simulink model "sgMdl_IO337_AnalogLoopback"  (R2024b)
settings: Solver=FixedStepAuto  StartTime=0.0  StopTime=inf  RelTol=1e-3
undefined symbols (not defined in the file): IO336, IO3xx, Pull, pull, up
libraries: speedgoatlib_fpga_analog_io x3, slrealtimeloglib x2, speedgoatlib_fpga x1
Description:
  | IO337 - Analog Loopback
settings Model: ModifiedByFormat=Speedgoat  SimulationMode=external  ExtModeTrigDuration=100000  Creator=Speedgoat  LastModifiedBy=Speedgoat
settings SolverCC: ConcurrentTasks=on  PositivePriorityOrder=on
settings DataIOCC: SaveFormat=StructureWithTime
settings OptimizationCC: BlockReduction=off  OptimizeBlockIOStorage=off  BufferReuse=off  ReuseModelBlockBuffer=off
settings DebuggingCC: UnderspecifiedInitializationDetection=Classic  MergeDetectMultiDrivingBlocksExec=none  TasksWithSamePriorityMsg=none
settings HardwareCC: ProdBitPerLong=64  ProdLongLongMode=on  ProdHWDeviceType=Intel->x86-64 (Linux 64)
settings ModelReferenceCC: EnableRefExpFcnMdlSchedulingChecks=on  PropagateSignalLabelsOutOfModel=off
settings RTWCC: Description=Speedgoat Real-Time Target Machine  SystemTargetFile=speedgoat.tlc  TemplateMakefile=slrealtime_default_tmf  PostCodeGenCommand=sg.model.build.makeCfg(bdroot, buildInfo);  Toolchain=Simulink Real-Time Toolchain  BuildConfiguration=Faster Runs  TargetLang=C++  GPUComputeCapability=3.5
settings SimulinkRealTimeTargetCC: SubcomponentCodeInterfacePackaging=Reusable function  InstructionSetFMA=off  LogToMDFFile=off  SLRTFileLogMaxRuns=10
settings ConfigComp: CovBoundaryAbsTol=1.0e-5

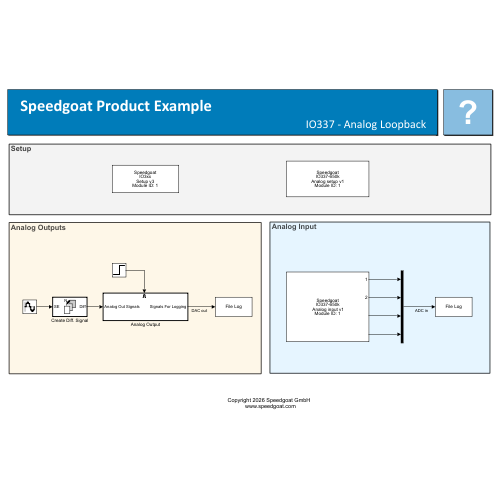
[thumbnail: Simulink's stored preview of the top-level diagram]
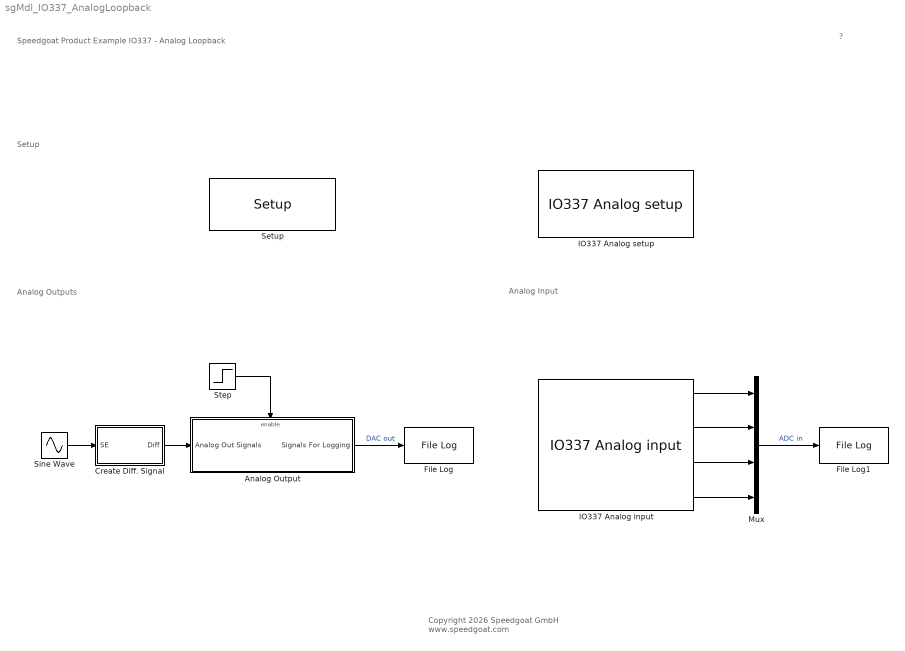
== system sgMdl_IO337_AnalogLoopback ==
  note: Analog Outputs
  note: Analog Input
  note: Setup
  note: Speedgoat Product Example
      | IO337 - Analog Loopback
  note: ?
  note: Copyright 2026 Speedgoat GmbH
      |  www.speedgoat.com
  Analog Output : Subsystem
  Create Diff. Signal : Subsystem  TreatAsAtomicUnit=on
  File Log : slrealtimeloglib/File Log  decimation=1  inputProcessing=Elements as channels (sample based)
  File Log1 : slrealtimeloglib/File Log  decimation=1  inputProcessing=Elements as channels (sample based)
  IO337 Analog input : speedgoatlib_fpga_analog_io/IO337/IO337 Analog input  id=1  parSampleTime=-1  pciSlot=[-1,-1]  parAiChannels=[1 2 3 4]  parAiChannelsStreamed=[1 2 3 4]  parAiTriggerMode=[2 2]  parAiReadPrevValue=0  parAiEnableFrame=0  parAdcCoupling=[1 1 1 1]  parAdcContSampling=0  parAdcDmaEnable=0  parAdcActiveDmaDevices=[1 1 1 1]  parAiFrameSize=100
      settings: SourceProductName=Analog IO
  IO337 Analog setup : speedgoatlib_fpga_analog_io/IO337/IO337 Analog setup  id=1  siteIdx=1  parEnableCodeModule1=off  parEnableCodeModule2=off  parEnableCodeModule3=off  parEnableCodeModule4=off  parEnableCodeModule5=off  parEnableCodeModule6=off  parEnableCodeModule7=off  parEnableCodeModule8=off  parAdcEnableIndividualTrigger=off  parAdcDisableSampleRead=off  parAdcTriggerMode1=Model Step  parAdcSampleRate1=1e5  parAdcDioTriggerChannel1=1  parAdcInternalTrigger1=<empty>  parAdcOversampling1=None  parAdcTriggerMode2=Model Step  parAdcSampleRate2=1e5  parAdcDioTriggerChannel2=1  parAdcInternalTrigger2=<empty>  parAdcOversampling2=None  parAdcTriggerMode3=Model Step  parAdcSampleRate3=1e5  parAdcDioTriggerChannel3=1  parAdcInternalTrigger3=<empty>  parAdcOversampling3=None  parAdcTriggerMode4=Model Step  parAdcSampleRate4=1e5  parAdcDioTriggerChannel4=1  parAdcInternalTrigger4=<empty>  parAdcOversampling4=None  parAdcReadPrevValueIndividualTrigger=off  parAdcEnableFrame=off  parAdcTriggerMode=Model Step  parAdcReadPrevValue=off  parAdcSampleRate=100e3  parAdcDioTriggerChannel=1  parAdcInternalTrigger=<empty>  parAdcOversampling=None  parAdcTriggerResolution=1e-08  parAdcSampleRateFrame=1e5  parAdcFrameSize=100  parAdcSampleTime=-1  parDacTriggerMode=Model Step  parDacInternalTrigger=<empty>  parDacDioTriggerChannel=1  parDacEnableFrame=on  dacUsesTimer=on  parDacFifoThreshold=100  parDacTriggerResolution=1e-08  parDacSampleRate=1e6  parDacFrameSize=1000  parDacSampleTime=-1  parAdcChannel1=on  parAdcChannel2=on  parAdcChannel3=on  parAdcChannel4=on  parAdcChannel5=off  parAdcChannel6=off  parAdcChannel7=off  parAdcChannel8=off  parAdcAutoCorrection=on  parDacChannel1=on  parDacChannel2=on  parDacChannel3=on  parDacChannel4=on  parDacChannel5=off  parDacChannel6=off  parDacChannel7=off  parDacChannel8=off  parDacChannel9=off  parDacChannel10=off  parDacChannel11=off  parDacChannel12=off  parDacChannel13=off  parDacChannel14=off  parDacChannel15=off  parDacChannel16=off  parDacChannel17=off  parDacChannel18=off  parDacChannel19=off  parDacChannel20=off  parDacChannel21=off  parDacChannel22=off  parDacChannel23=off  parDacChannel24=off  parDacChannel25=off  parDacChannel26=off  parDacChannel27=off  parDacChannel28=off  parDacChannel29=off  parDacChannel30=off  parDacChannel31=off  parDacChannel32=off  parDacEnbIndividualSettings=on  parDacRangeCommon=+-10 V  parDacInitValueCommon=0  parDacResetCommon=on  parDacRange1=+-10 V  parDacInitValue1=0  parDacReset1=off  parDacRange2=+-10 V  parDacInitValue2=0  parDacReset2=off  parDacRange3=+-10 V  parDacInitValue3=0  parDacReset3=off  parDacRange4=+-10 V  parDacInitValue4=0  parDacReset4=off  parDacRange5=+-10 V  parDacInitValue5=0  parDacReset5=on  parDacRange6=+-10 V  parDacInitValue6=0  parDacReset6=on  parDacRange7=+-10 V  parDacInitValue7=0  parDacReset7=on  parDacRange8=+-10 V  parDacInitValue8=0  parDacReset8=on  parDacRange9=+-10 V  parDacInitValue9=0  parDacReset9=on  parDacRange10=+-10 V  parDacInitValue10=0  parDacReset10=on  parDacRange11=+-10 V  parDacInitValue11=0  parDacReset11=on  parDacRange12=+-10 V  parDacInitValue12=0  parDacReset12=on  parDacRange13=+-10 V  parDacInitValue13=0  parDacReset13=on  parDacRange14=+-10 V  parDacInitValue14=0  parDacReset14=on  parDacRange15=+-10 V  parDacInitValue15=0  parDacReset15=on  parDacRange16=+-10 V  parDacInitValue16=0  parDacReset16=on  parDacRange17=+-10 V  parDacInitValue17=0  parDacReset17=on  parDacRange18=+-10 V  parDacInitValue18=0  parDacReset18=on  parDacRange19=+-10 V  parDacInitValue19=0  parDacReset19=on  parDacRange20=+-10 V  parDacInitValue20=0  parDacReset20=on  parDacRange21=+-10 V  parDacInitValue21=0  parDacReset21=on  parDacRange22=+-10 V  parDacInitValue22=0  parDacReset22=on  parDacRange23=+-10 V  parDacInitValue23=0  parDacReset23=on  parDacRange24=+-10 V  parDacInitValue24=0  parDacReset24=on  parDacRange25=+-10 V  parDacInitValue25=0  parDacReset25=on  parDacRange26=+-10 V  parDacInitValue26=0  parDacReset26=on  parDacRange27=+-10 V  parDacInitValue27=0  parDacReset27=on  parDacRange28=+-10 V  parDacInitValue28=0  parDacReset28=on  parDacRange29=+-10 V  parDacInitValue29=0  parDacReset29=on  parDacRange30=+-10 V  parDacInitValue30=0  parDacReset30=on  parDacRange31=+-10 V  parDacInitValue31=0  parDacReset31=on  parDacRange32=+-10 V  parDacInitValue32=0  parDacReset32=on  parDacAutoCorrection=on
      settings: SourceProductName=Analog IO
  Mux : Mux
  Setup : speedgoatlib_fpga/Setup/Setup  board=Please select...  id=1  pciSlot=-1  device_id=1  bitstreamFilePath=C:\SVN\speedgoatlib\releases\10.0.0\product_examples\IO337  bitstreamFile=Please select...  fpgaFreq=[100000000 125000000]  enableDma=on  rearEnb_1=off  rearIO_1=IO3xx-21  rearEnb_2=off  rearIO_2=None  ProgSpiFlash=off  ProgBPIFlash=off  useFpgaDmaController=off  dmaTrigDropdown=Model Step  dmaTrigSelect=0  dmaStopOnOverload=on  dmaModeSequential=on  dmaModeParallel=off  PullRPort15=pull-up 3.3V  PullRPort31=pull-up 3.3V  PullRPort47=pull-up 3.3V  PullRPort63=pull-up 3.3V  diffLineTermination_1=on  diffLineTermination_2=on  diffLineTermination_3=on  diffLineTermination_4=on  diffLineTermination_5=on  diffLineTermination_6=on  diffLineTermination_7=on  diffLineTermination_8=on  diffLineTermination_9=on  diffLineTermination_10=on  diffLineTermination_11=on  diffLineTermination_12=on  diffLineTermination_13=on  diffLineTermination_14=on  diffLineTermination_15=on  diffLineTermination_16=on  diffLineTermination_17=on  diffLineTermination_18=on  diffLineTermination_19=on  diffLineTermination_20=on  diffLineTermination_21=on  diffLineTermination_22=on  diffLineTermination_23=on  diffLineTermination_24=on  diffLineTermination_25=on  diffLineTermination_26=on  diffLineTermination_27=on  diffLineTermination_28=on  diffLineTermination_29=on  diffLineTermination_30=on  diffLineTermination_31=on  diffLineTermination_32=on  ioVoltageDropDown1=3.3V  pullResistorDropDown1_1=Pull-up  pullResistorDropDown1_2=Pull-up  pullResistorDropDown1_3=Pull-up  pullResistorDropDown1_4=Pull-up  pullResistorDropDown1_5=Pull-up  pullResistorDropDown1_6=Pull-up  pullResistorDropDown1_7=Pull-up  pullResistorDropDown1_8=Pull-up  ttlIsImplementedCheckBox1=off  pullResistorDropDown2=Pull-up  ioVoltageDropDown2=3.3V  ttlIsImplementedCheckBox2=off  pullResistorDropDown3=Pull-up  ioVoltageDropDown3=3.3V  ttlIsImplementedCheckBox3=off  pullResistorDropDown4=Pull-up  ioVoltageDropDown4=3.3V  ttlIsImplementedCheckBox4=off  pullResistorDropDown5=Pull-up  ioVoltageDropDown5=3.3V  ttlIsImplementedCheckBox5=off  pullResistorDropDown6=Pull-up  ioVoltageDropDown6=3.3V  ttlIsImplementedCheckBox6=off  pullResistorDropDown7=Pull-up  ioVoltageDropDown7=3.3V  ttlIsImplementedCheckBox7=off  pullResistorDropDown8=Pull-up  ioVoltageDropDown8=3.3V  ttlIsImplementedCheckBox8=off  terminationCheckBox1=off  terminationCheckBox2=off  terminationCheckBox3=off  terminationCheckBox4=off  diffIsImplementedCheckBox1=off  terminationCheckBox5=off  terminationCheckBox6=off  terminationCheckBox7=off  terminationCheckBox8=off  diffIsImplementedCheckBox2=off  terminationCheckBox9=off  terminationCheckBox10=off  terminationCheckBox11=off  terminationCheckBox12=off  diffIsImplementedCheckBox3=off  terminationCheckBox13=off  terminationCheckBox14=off  terminationCheckBox15=off  terminationCheckBox16=off  diffIsImplementedCheckBox4=off  terminationCheckBox17=off  terminationCheckBox18=off  terminationCheckBox19=off  terminationCheckBox20=off  diffIsImplementedCheckBox5=off  terminationCheckBox21=off  terminationCheckBox22=off  terminationCheckBox23=off  terminationCheckBox24=off  diffIsImplementedCheckBox6=off  terminationCheckBox25=off  terminationCheckBox26=off  terminationCheckBox27=off  terminationCheckBox28=off  diffIsImplementedCheckBox7=off  terminationCheckBox29=off  terminationCheckBox30=off  terminationCheckBox31=off  terminationCheckBox32=off  diffIsImplementedCheckBox8=off  PullRPort0_1=pull-up  VioPort0_1=3.3V  PullRPort1_1=pull-up  VioPort1_1=3.3V  PullRPort2_1=pull-up  VioPort2_1=3.3V  PullRPort3_1=pull-up  VioPort3_1=3.3V  PullRPort4_1=pull-up  VioPort4_1=3.3V  PullRPort5_1=pull-up  VioPort5_1=3.3V  PullRPort6_1=pull-up  VioPort6_1=3.3V  diffLineTermination_rear1_1=on  diffLineTermination_rear1_2=on  diffLineTermination_rear1_3=on  diffLineTermination_rear1_4=on  diffLineTermination_rear1_5=on  diffLineTermination_rear1_6=on  diffLineTermination_rear1_7=on  diffLineTermination_rear1_8=on  PullRPort0_2=pull-up  VioPort0_2=3.3V  PullRPort1_2=pull-up  VioPort1_2=3.3V  PullRPort2_2=pull-up  VioPort2_2=3.3V  PullRPort3_2=pull-up  VioPort3_2=3.3V  PullRPort4_2=pull-up  VioPort4_2=3.3V  PullRPort5_2=pull-up  VioPort5_2=3.3V  PullRPort6_2=pull-up  VioPort6_2=3.3V  diffLineTermination_rear2_1=on  diffLineTermination_rear2_2=on  diffLineTermination_rear2_3=on  diffLineTermination_rear2_4=on  diffLineTermination_rear2_5=on  diffLineTermination_rear2_6=on  diffLineTermination_rear2_7=on  diffLineTermination_rear2_8=on
      settings: SourceProductName=IO3xx
  Sine Wave : Sin  Amplitude=[1,2]  Frequency=10*2*pi  SampleTime=1e-3
  Step : Step  Time=0.5  SampleTime=1e-3
  wires:
  Mux/1 -> File Log1/1  "ADC in"
  IO337 Analog input/1 -> Mux/1
  IO337 Analog input/2 -> Mux/2
  Sine Wave/1 -> Create Diff. Signal/1(SE)
  Analog Output/1(Signals For Logging) -> File Log/1  "DAC out"
  Step/1 -> Analog Output/Enable
  Create Diff. Signal/1(Diff) -> Analog Output/1(Analog Out Signals)
  IO337 Analog input/3 -> Mux/3
  IO337 Analog input/4 -> Mux/4

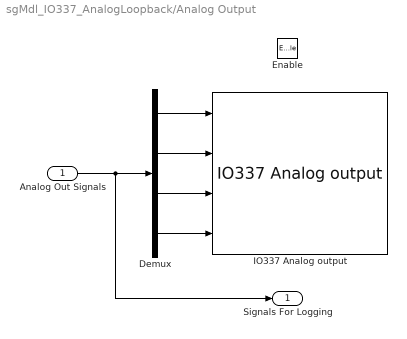
== system sgMdl_IO337_AnalogLoopback/Analog Output ==
  Analog Out Signals : Inport
  Enable : EnablePort
  Demux : Demux
  IO337 Analog output : speedgoatlib_fpga_analog_io/IO337/IO337 Analog output  id=1  parSampleTime=-1  pciSlot=[-1,-1]  board=IO336-325k  parAoChannels=[1 2 3 4]  parAoVoltageRange=[1 1 1 1]  parDacOverRange=[0 0 0 0 0 0 0 0]  parAoInitValues=[0 0 0 0]  parAoReset=[0 0 0 0]  parDacSyncOut=1  parAoEnableFrame=0  parDacActiveDmaDevices=[1 1 1 1]  parDacDmaLatency=2  parAoFrameSize=1000
      settings: SourceProductName=Analog IO
  Signals For Logging : Outport
  wires:
  Analog Out Signals/1 -> Signals For Logging/1, Demux/1
  Demux/2 -> IO337 Analog output/2
  Demux/3 -> IO337 Analog output/3
  Demux/1 -> IO337 Analog output/1
  Demux/4 -> IO337 Analog output/4

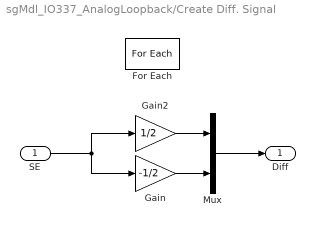
== system sgMdl_IO337_AnalogLoopback/Create Diff. Signal ==
  SE : Inport  Partition=on  PartitionDimension=1  PartitionWidth=1  PartitionOffset=0
  For Each : ForEach  DisableCoverage=on
  Gain : Gain  Gain=-1/2
  Gain2 : Gain  Gain=1/2
  Mux : Mux  Inputs=2
  Diff : Outport  ConcatenationDimension=1
  wires:
  Gain2/1 -> Mux/1
  Gain/1 -> Mux/2
  SE/1 -> Gain/1, Gain2/1
  Mux/1 -> Diff/1
